simulink model "Copy_of_BasePlant"  (R2021b)
settings: Solver=VariableStepAuto  StartTime=0.0  StopTime=10.0  RelTol=1e-3
undefined symbols (not defined in the file): cmFuel_cmL, g, m_dot, m_iFuel, W_lander
libraries: shared6dof x1
settings Model: Creator=josepfamador  LastModifiedBy=josepfamador
settings DebuggingCC: SignalRangeChecking=warning

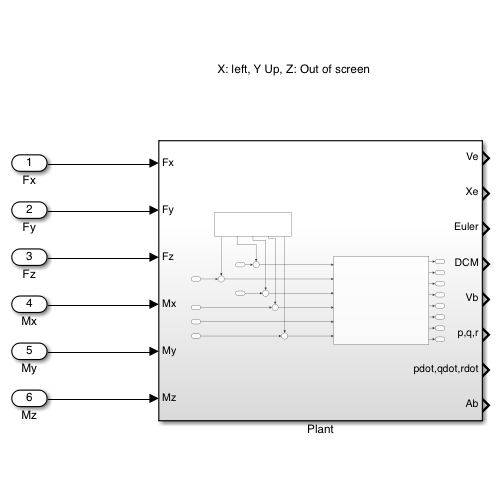
[thumbnail: Simulink's stored preview of the top-level diagram]
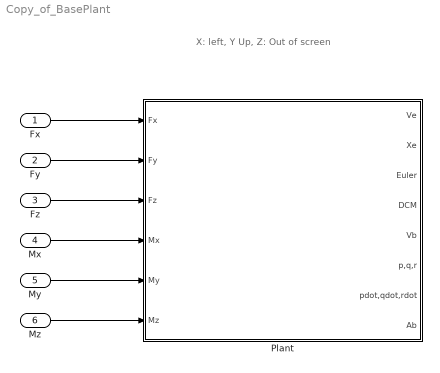
== system Copy_of_BasePlant ==
  note: X: left, Y Up, Z: Out of screen
  Fx : Inport
  Fy : Inport  Port=2
  Fz : Inport  Port=3
  Mx : Inport  Port=4
  My : Inport  Port=5
  Mz : Inport  Port=6
  Plant : Subsystem
  wires:
  Fx/1 -> Plant/1(Fx)
  Fy/1 -> Plant/2(Fy)
  Fz/1 -> Plant/3(Fz)
  Mx/1 -> Plant/4(Mx)
  My/1 -> Plant/5(My)
  Mz/1 -> Plant/6(Mz)

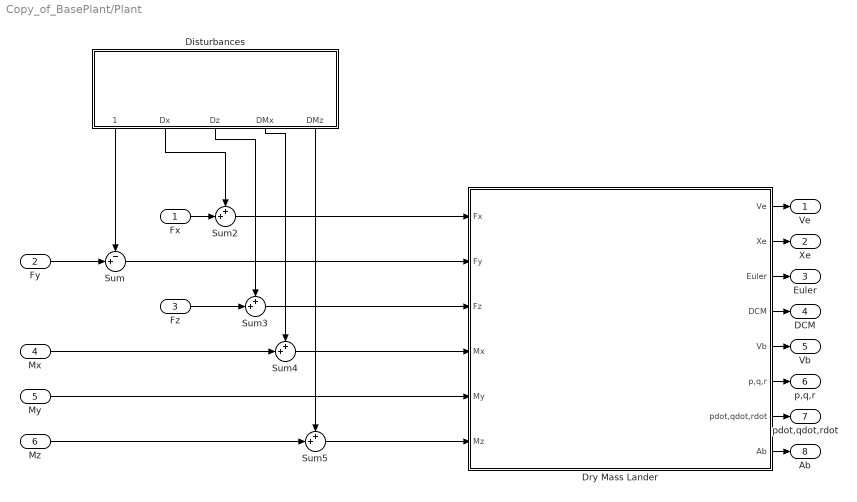
== system Copy_of_BasePlant/Plant ==
  Fx : Inport
  Fy : Inport  Port=2
  Fz : Inport  Port=3
  Mx : Inport  Port=4
  My : Inport  Port=5
  Mz : Inport  Port=6
  Disturbances : Subsystem
  Dry Mass Lander : Subsystem
  Sum : Sum  Inputs=-+|
  Sum{2..5} (4 alike) : Sum  Inputs=++|
  Ve : Outport
  Xe : Outport  Port=2
  Euler : Outport  Port=3
  DCM : Outport  Port=4
  Vb : Outport  Port=5
  p,q,r : Outport  Port=6
  pdot,qdot,rdot : Outport  Port=7
  Ab : Outport  Port=8
  wires:
  Dry Mass Lander/4(DCM) -> DCM/1
  Disturbances/3(Dz) -> Sum3/1
  Dry Mass Lander/2(Xe) -> Xe/1
  Dry Mass Lander/5(Vb) -> Vb/1
  My/1 -> Dry Mass Lander/5(My)
  Disturbances/4(DMx) -> Sum4/1
  Dry Mass Lander/6(p,q,r) -> p,q,r/1
  Sum4/1 -> Dry Mass Lander/4(Mx)
  Dry Mass Lander/1(Ve) -> Ve/1
  Disturbances/2(Dx) -> Sum2/1
  Fy/1 -> Sum/2
  Sum3/1 -> Dry Mass Lander/3(Fz)
  Sum2/1 -> Dry Mass Lander/1(Fx)
  Fx/1 -> Sum2/2
  Disturbances/5(DMz) -> Sum5/1
  Disturbances/1(Weight_Fuel) -> Sum/1
  Dry Mass Lander/3(Euler) -> Euler/1
  Fz/1 -> Sum3/2
  Sum/1 -> Dry Mass Lander/2(Fy)
  Dry Mass Lander/7(pdot,qdot,rdot) -> pdot,qdot,rdot/1
  Dry Mass Lander/8(Ab) -> Ab/1
  Mx/1 -> Sum4/2
  Mz/1 -> Sum5/2
  Sum5/1 -> Dry Mass Lander/6(Mz)

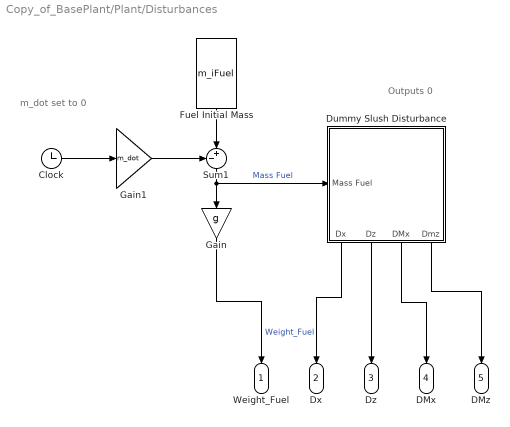
== system Copy_of_BasePlant/Plant/Disturbances ==
  note: m_dot set to 0
  note: Outputs 0
  Clock : Clock
  Dummy Slush Disturbance : Subsystem
      settings: PortSchema="{\"entries\":[{\"content\":{\"sides\":[{\"content\":{\"connectorIds\":[]},\"type\":\"ConnectorPlacement.EquallySpacedRectSide\",\"uuid\":\"6993c7b3-d1aa-4729-9312-d218de701469\"},{\"content\":{\"connectorIds\":[\"Out1\",\"Out2\",\"Out3\",\"Out4\"],\"side\":\"RIGHT\"},\"type\":\"ConnectorPlacement.EquallySpacedRectSide\",\"uuid\":\"b34002d0-f017-4c93-94f6-1c57307a66f4\"},{\"content\":{\"connectorIds\":[\"In1\"],\"side\":\"TOP\"},\"type\":\"ConnectorPlacement.EquallySpacedRectSide\",\"uuid\":\"9236c70f-177a-4213-a876-d93db0a147ef\"}]},\"type\":\"ConnectorPlacement.EquallySpacedConnector\",\"uuid\":\"952db336-e8ce-4b54-9b0c-19bfd8ec6529\"}],\"packageUris\":[\"http://schema.mathworks.com/mf0/Connector/R2020b\"],\"version\":\"1.0\"}"
  Fuel Initial Mass : Constant  Value=m_iFuel
  Gain : Gain  Gain=g
  Gain1 : Gain  Gain=m_dot
  Sum1 : Sum  Inputs=-+|
  Weight_Fuel : Outport
  Dx : Outport  Port=2
  Dz : Outport  Port=3
  DMx : Outport  Port=4
  DMz : Outport  Port=5
  wires:
  Dummy Slush Disturbance/4(Dmz) -> DMz/1
  Dummy Slush Disturbance/1(Dx) -> Dx/1
  Dummy Slush Disturbance/2(Dz) -> Dz/1
  Clock/1 -> Gain1/1
  Gain1/1 -> Sum1/1
  Gain/1 -> Weight_Fuel/1  "Weight_Fuel"
  Sum1/1 -> Gain/1, Dummy Slush Disturbance/1(Mass Fuel)  "Mass Fuel"
  Dummy Slush Disturbance/3(DMx) -> DMx/1
  Fuel Initial Mass/1 -> Sum1/2

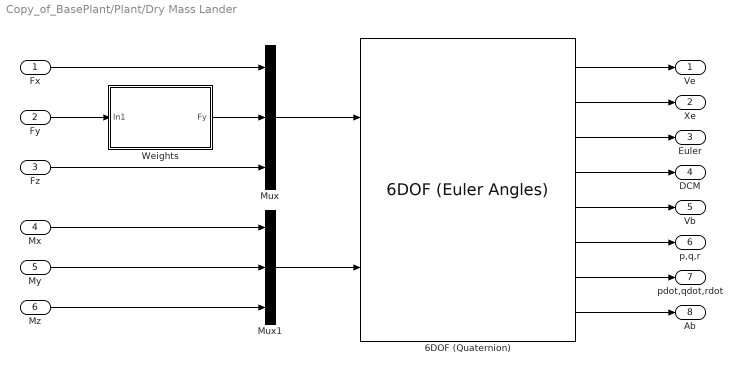
== system Copy_of_BasePlant/Plant/Dry Mass Lander ==
  Fx : Inport
  Fy : Inport  Port=2
  Fz : Inport  Port=3
  Mx : Inport  Port=4
  My : Inport  Port=5
  Mz : Inport  Port=6
  6DOF (Quaternion) : shared6dof/6DOF (Euler Angles)  units=Metric (MKS)  mtype=Fixed  rep=Quaternion  xme_0=[0 0 0]  Vm_0=[0 0 0]  eul_0=[0 0 0]  pm_0=[0 0 0]  mass_0=1.0  mass_e=0.5  mass_f=2.0  inertia=eye(3)  inertia_e=eye(3)  inertia_f=2*eye(3)  k_quat=1.0  vre_flag=on  abi_flag=off  aMode=0  xme_statename=''  Vm_statename=''  eul_statename=''  quat_statename=''  pm_statename=''  mass_statename=''
      settings: SourceProductBaseCode=AE,PW,DR,MT,UV,VE
  Mux : Mux  Inputs=3
  Mux1 : Mux  Inputs=3
  Weights : Subsystem
  Ve : Outport
  Xe : Outport  Port=2
  Euler : Outport  Port=3
  DCM : Outport  Port=4
  Vb : Outport  Port=5
  p,q,r : Outport  Port=6
  pdot,qdot,rdot : Outport  Port=7
  Ab : Outport  Port=8
  wires:
  6DOF (Quaternion)/7 -> pdot,qdot,rdot/1
  6DOF (Quaternion)/1 -> Ve/1
  6DOF (Quaternion)/2 -> Xe/1
  6DOF (Quaternion)/4 -> DCM/1
  6DOF (Quaternion)/5 -> Vb/1
  Mux/1 -> 6DOF (Quaternion)/1
  Mx/1 -> Mux1/1
  Mux1/1 -> 6DOF (Quaternion)/2
  Weights/1(Fy) -> Mux/2
  6DOF (Quaternion)/6 -> p,q,r/1
  Fz/1 -> Mux/3
  6DOF (Quaternion)/3 -> Euler/1
  6DOF (Quaternion)/8 -> Ab/1
  Fx/1 -> Mux/1
  Mz/1 -> Mux1/3
  Fy/1 -> Weights/1(In1)
  My/1 -> Mux1/2

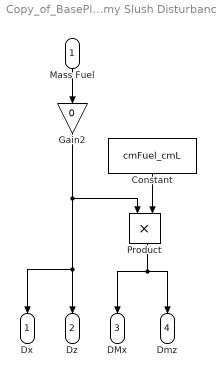
== system Copy_of_BasePlant/Plant/Disturbances/Dummy Slush Disturbance ==
  Mass Fuel : Inport
  Constant : Constant  Value=cmFuel_cmL
  Gain2 : Gain  Gain=0
  Product : Product
  Dx : Outport
  Dz : Outport  Port=2
  DMx : Outport  Port=3
  Dmz : Outport  Port=4
  wires:
  Constant/1 -> Product/2
  Mass Fuel/1 -> Gain2/1
  Gain2/1 -> Dz/1, Dx/1, Product/1
  Product/1 -> Dmz/1, DMx/1

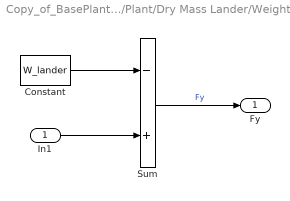
== system Copy_of_BasePlant/Plant/Dry Mass Lander/Weights ==
  In1 : Inport
  Constant : Constant  Value=W_lander
  Sum : Sum  Inputs=-+
  Fy : Outport
  wires:
  Sum/1 -> Fy/1  "Fy"
  In1/1 -> Sum/2
  Constant/1 -> Sum/1
